simulink model "uz_dac_spi_interface"  (R2023a)
settings: Solver=FixedStepDiscrete  StartTime=0.0  StopTime=1000/100e6  RelTol=1e-3
libraries: hdlsllib x152, simulink x2
settings Model: DataTypeOverride=Off  Creator=ts  LastModifiedBy=ts
settings SolverCC: AlgebraicLoopSolver=TrustRegion
settings DataIOCC: LimitDataPoints=on  SaveOutput=off  SaveTime=off
settings OptimizationCC: BlockReduction=off  ConditionallyExecuteInputs=off  DefaultParameterBehavior=Inlined  LifeSpan=inf
settings DebuggingCC: AlgebraicLoopMsg=error  SingleTaskRateTransMsg=error  UnconnectedInputMsg=warning  UnconnectedOutputMsg=warning  UnconnectedLineMsg=warning  AllowSymbolicDim=off  StrictBusMsg=ErrorOnBusTreatedAsVector  SFUnexpectedBacktrackingDiag=warning  SFNoUnconditionalDefaultTransitionDiag=warning  SFExecutionAtInitializationDiag=none  ArithmeticOperatorsInVariantConditions=warning
settings HardwareCC: ProdBitPerPointer=32  ProdBitPerSizeT=32  ProdBitPerPtrDiffT=32  ProdLargestAtomicFloat=None  ProdIntDivRoundTo=Undefined  ProdEndianess=Unspecified  ProdWordSize=32  ProdHWDeviceType=ASIC/FPGA->ASIC/FPGA  ProdEqTarget=off
settings ModelReferenceCC: EnableRefExpFcnMdlSchedulingChecks=on
settings SFSimCC: SimUseLocalCustomCode=off  CustomCodeUndefinedFunction=UseInterfaceOnly
settings RTWCC: RTWUseLocalCustomCode=off
settings CodeAppCC: StateflowObjectComments=on
settings GRTTargetCC: TargetLangStandard=C89/C90 (ANSI)
settings ConfigComp: CovScope=ReferencedModels  CovMetricSettings=dw  CovSaveCumulativeToWorkspaceVar=on  CovSaveSingleToWorkspaceVar=on  CovExternalEMLEnable=off  CovSFcnEnable=off

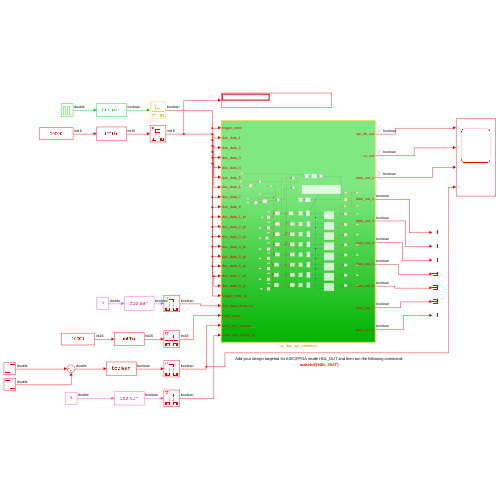
[thumbnail: Simulink's stored preview of the top-level diagram]
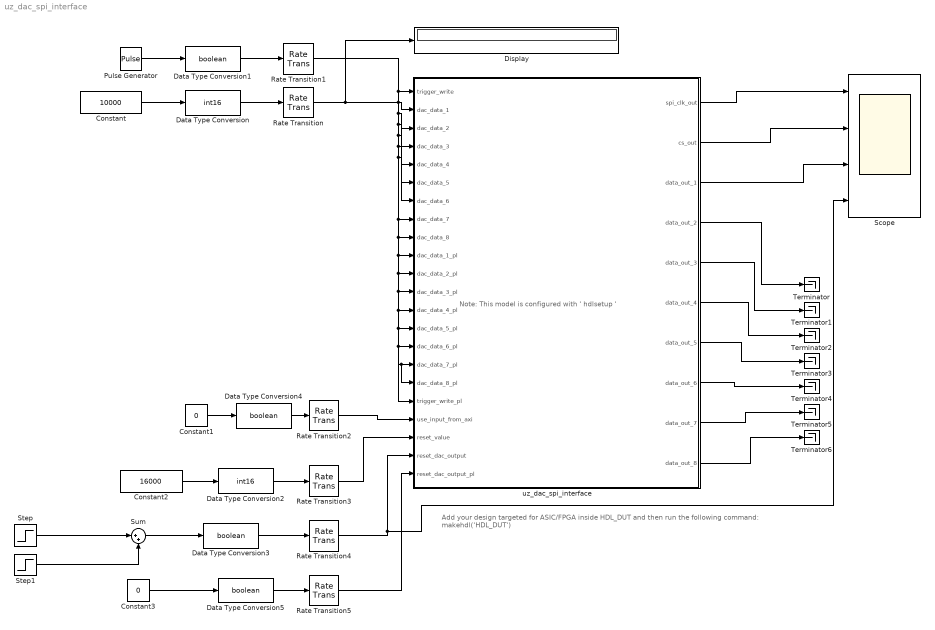
== system uz_dac_spi_interface ==
  note: Note: This model is configured with ' hdlsetup '
  note: Add your design targeted for ASIC/FPGA inside HDL_DUT and then run the following command:
      | makehdl('HDL_DUT')
  Constant : Constant  Value=10000  OutDataTypeStr=int16  SampleTime=1/100e6
  Constant1 : Constant  Value=0
  Constant2 : Constant  Value=16000  OutDataTypeStr=int16  SampleTime=1/100e6
  Constant3 : Constant  Value=0
  Data Type Conversion : DataTypeConversion  OutDataTypeStr=int16  SaturateOnIntegerOverflow=off  RndMeth=Floor
  Data Type Conversion{1,3..5} (4 alike) : DataTypeConversion  OutDataTypeStr=boolean  SaturateOnIntegerOverflow=off  RndMeth=Floor
  Data Type Conversion2 : DataTypeConversion  OutDataTypeStr=int16  SaturateOnIntegerOverflow=off  RndMeth=Floor
  Display : Display
      settings: Format=binary (Stored Integer)
  Pulse Generator : DiscretePulseGenerator  PulseType=Time based  Period=200/100e6  PulseWidth=10
  Rate Transition{,1..5} (6 alike) : RateTransition  OutPortSampleTime=1/100e6
  Scope : Scope  NumInputPorts=4
  Step : Step  Time=240/100e6
  Step1 : Step  Time=500/100e6  After=-1
  Sum : Sum  Inputs=|++
  Terminator{,1..6} (7 alike) : Terminator
  uz_dac_spi_interface : Subsystem  TreatAsAtomicUnit=on
  wires:
  Constant/1 -> Data Type Conversion/1
  uz_dac_spi_interface/3(data_out_1) -> Scope/3
  Data Type Conversion/1 -> Rate Transition/1
  Rate Transition/1 -> Display/1, uz_dac_spi_interface/17(dac_data_8_pl), uz_dac_spi_interface/16(dac_data_7_pl), uz_dac_spi_interface/15(dac_data_6_pl), uz_dac_spi_interface/14(dac_data_5_pl), uz_dac_spi_interface/13(dac_data_4_pl), uz_dac_spi_interface/12(dac_data_3_pl), uz_dac_spi_interface/11(dac_data_2_pl), uz_dac_spi_interface/10(dac_data_1_pl), uz_dac_spi_interface/9(dac_data_8), uz_dac_spi_interface/8(dac_data_7), uz_dac_spi_interface/7(dac_data_6), uz_dac_spi_interface/6(dac_data_5), uz_dac_spi_interface/5(dac_data_4), uz_dac_spi_interface/4(dac_data_3), uz_dac_spi_interface/3(dac_data_2), uz_dac_spi_interface/2(dac_data_1)
  uz_dac_spi_interface/2(cs_out) -> Scope/2
  uz_dac_spi_interface/1(spi_clk_out) -> Scope/1
  Rate Transition1/1 -> uz_dac_spi_interface/1(trigger_write), uz_dac_spi_interface/18(trigger_write_pl)
  Data Type Conversion1/1 -> Rate Transition1/1
  Pulse Generator/1 -> Data Type Conversion1/1
  Rate Transition2/1 -> uz_dac_spi_interface/19(use_input_from_axi)
  Constant1/1 -> Data Type Conversion4/1
  uz_dac_spi_interface/4(data_out_2) -> Terminator/1
  uz_dac_spi_interface/5(data_out_3) -> Terminator1/1
  uz_dac_spi_interface/6(data_out_4) -> Terminator2/1
  uz_dac_spi_interface/7(data_out_5) -> Terminator3/1
  uz_dac_spi_interface/8(data_out_6) -> Terminator4/1
  uz_dac_spi_interface/9(data_out_7) -> Terminator5/1
  uz_dac_spi_interface/10(data_out_8) -> Terminator6/1
  Constant2/1 -> Data Type Conversion2/1
  Data Type Conversion2/1 -> Rate Transition3/1
  Rate Transition3/1 -> uz_dac_spi_interface/20(reset_value)
  Data Type Conversion3/1 -> Rate Transition4/1
  Constant3/1 -> Data Type Conversion5/1
  Rate Transition5/1 -> uz_dac_spi_interface/22(reset_dac_output_pl)
  Data Type Conversion4/1 -> Rate Transition2/1
  Data Type Conversion5/1 -> Rate Transition5/1
  Rate Transition4/1 -> Scope/4, uz_dac_spi_interface/21(reset_dac_output)
  Sum/1 -> Data Type Conversion3/1
  Step/1 -> Sum/1
  Step1/1 -> Sum/2

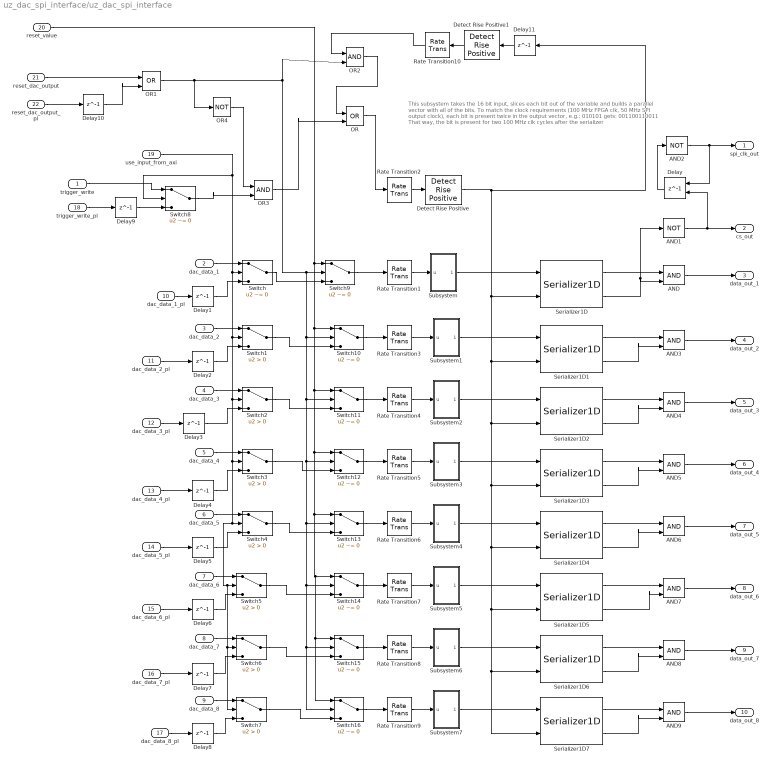
== system uz_dac_spi_interface/uz_dac_spi_interface ==
  note: This subsystem takes the 16 bit input, slices each bit out of the variable and builds a parallel vector with all of the bits.
      | To match the clock requirements (100 MHz FPGA clk, 50 MHz SPI output clock), each bit is present twice in the output vector, e.g.:
      | 010101 gets:
      | 001100110011
      | That way, the bit is present for two 100 MHz clk cycles after the serializer
  trigger_write : Inport
  dac_data_1 : Inport  Port=2
  dac_data_2 : Inport  Port=3
  dac_data_3 : Inport  Port=4
  dac_data_4 : Inport  Port=5
  dac_data_5 : Inport  Port=6
  dac_data_6 : Inport  Port=7
  dac_data_7 : Inport  Port=8
  dac_data_8 : Inport  Port=9
  dac_data_1_pl : Inport  Port=10
  dac_data_2_pl : Inport  Port=11
  dac_data_3_pl : Inport  Port=12
  dac_data_4_pl : Inport  Port=13
  dac_data_5_pl : Inport  Port=14
  dac_data_6_pl : Inport  Port=15
  dac_data_7_pl : Inport  Port=16
  dac_data_8_pl : Inport  Port=17
  trigger_write_pl : Inport  Port=18
  use_input_from_axi : Inport  Port=19
  reset_value : Inport  Port=20
  reset_dac_output : Inport  Port=21
  reset_dac_output_pl : Inport  Port=22
  AND{,3..9} (8 alike) : Logic  IconShape=distinctive  AllPortsSameDT=off  OutDataTypeStr=boolean
  AND1 : Logic  Operator=NOT  IconShape=distinctive  AllPortsSameDT=off  OutDataTypeStr=boolean
  AND2 : Logic  Operator=NOT  IconShape=distinctive  AllPortsSameDT=off  OutDataTypeStr=boolean
  Delay : Delay  DelayLength=1  InitialCondition=1  ExternalReset=Level
      settings: InputPortMap=u0,r5
  Delay{1..11} (11 alike) : Delay  DelayLength=1
  Detect Rise Positive : simulink/Logic and Bit Operations/Detect Rise Positive  vinit=0  OutDataTypeStr=boolean
  Detect Rise Positive1 : simulink/Logic and Bit Operations/Detect Rise Positive  vinit=0  OutDataTypeStr=boolean
  OR : Logic  Operator=OR  IconShape=distinctive  AllPortsSameDT=off  OutDataTypeStr=boolean
  OR1 : Logic  Operator=OR  IconShape=distinctive  AllPortsSameDT=off  OutDataTypeStr=boolean
  OR2 : Logic  IconShape=distinctive  AllPortsSameDT=off  OutDataTypeStr=boolean
  OR3 : Logic  IconShape=distinctive  AllPortsSameDT=off  OutDataTypeStr=boolean
  OR4 : Logic  Operator=NOT  IconShape=distinctive  AllPortsSameDT=off  OutDataTypeStr=boolean
  Rate Transition{1..9} (9 alike) : RateTransition  OutPortSampleTime=32/100e6
  Rate Transition10 : RateTransition
  Serializer1D{,1..7} (8 alike) : hdlsllib/HDL Operations/Serializer1D  Ratio=32  IdleCycles=0  validIn=on  startOut=off  validOut=on  inputDataDimensions=-1  inputSampleTime=-1  inputSignalType=auto
  Subsystem : Subsystem
  Subsystem1 : Subsystem
  Subsystem2 : Subsystem
  Subsystem3 : Subsystem
  Subsystem4 : Subsystem
  Subsystem5 : Subsystem
  Subsystem6 : Subsystem
  Subsystem7 : Subsystem
  Switch{,8..16} (10 alike) : Switch  Criteria=u2 ~= 0  SaturateOnIntegerOverflow=off  InputSameDT=off
  Switch{1..7} (7 alike) : Switch  Criteria=u2 > Threshold  SaturateOnIntegerOverflow=off  InputSameDT=off
  spi_clk_out : Outport
  cs_out : Outport  Port=2
  data_out_1 : Outport  Port=3  VectorParamsAs1DForOutWhenUnconnected=off
  data_out_2 : Outport  Port=4  VectorParamsAs1DForOutWhenUnconnected=off
  data_out_3 : Outport  Port=5  VectorParamsAs1DForOutWhenUnconnected=off
  data_out_4 : Outport  Port=6  VectorParamsAs1DForOutWhenUnconnected=off
  data_out_5 : Outport  Port=7  VectorParamsAs1DForOutWhenUnconnected=off
  data_out_6 : Outport  Port=8  VectorParamsAs1DForOutWhenUnconnected=off
  data_out_7 : Outport  Port=9  VectorParamsAs1DForOutWhenUnconnected=off
  data_out_8 : Outport  Port=10  VectorParamsAs1DForOutWhenUnconnected=off
  wires:
  AND/1 -> data_out_1/1
  Serializer1D/2 -> AND1/1, AND/2
  trigger_write/1 -> Switch8/1
  Detect Rise Positive/1 -> Serializer1D6/2, Serializer1D7/2, Serializer1D5/2, Serializer1D4/2, Serializer1D3/2, Serializer1D2/2, Serializer1D1/2, Serializer1D/2, Delay11/1
  Serializer1D/1 -> AND/1
  AND1/1 -> cs_out/1, Delay/2
  AND2/1 -> Delay/1, spi_clk_out/1
  Delay/1 -> AND2/1
  Rate Transition2/1 -> Detect Rise Positive/1
  Rate Transition1/1 -> Subsystem/1(u)
  Subsystem/1(Out1) -> Serializer1D/1
  Subsystem2/1(Out1) -> Serializer1D2/1
  Subsystem3/1(Out1) -> Serializer1D3/1
  Subsystem1/1(Out1) -> Serializer1D1/1
  Subsystem4/1(Out1) -> Serializer1D4/1
  Rate Transition3/1 -> Subsystem1/1(u)
  Rate Transition4/1 -> Subsystem2/1(u)
  Rate Transition5/1 -> Subsystem3/1(u)
  Rate Transition6/1 -> Subsystem4/1(u)
  Subsystem7/1(Out1) -> Serializer1D7/1
  Subsystem5/1(Out1) -> Serializer1D5/1
  Subsystem6/1(Out1) -> Serializer1D6/1
  Rate Transition7/1 -> Subsystem5/1(u)
  Rate Transition8/1 -> Subsystem6/1(u)
  Rate Transition9/1 -> Subsystem7/1(u)
  AND3/1 -> data_out_2/1
  Serializer1D1/1 -> AND3/1
  Serializer1D1/2 -> AND3/2
  AND4/1 -> data_out_3/1
  AND5/1 -> data_out_4/1
  AND6/1 -> data_out_5/1
  AND7/1 -> data_out_6/1
  AND8/1 -> data_out_7/1
  AND9/1 -> data_out_8/1
  Serializer1D2/1 -> AND4/1
  Serializer1D2/2 -> AND4/2
  Serializer1D3/1 -> AND5/1
  Serializer1D3/2 -> AND5/2
  Serializer1D4/1 -> AND6/1
  Serializer1D4/2 -> AND6/2
  Serializer1D5/1 -> AND7/1
  Serializer1D5/2 -> AND7/2
  Serializer1D6/1 -> AND8/1
  Serializer1D6/2 -> AND8/2
  Serializer1D7/1 -> AND9/1
  Serializer1D7/2 -> AND9/2
  dac_data_1/1 -> Switch/1
  dac_data_3/1 -> Switch2/1
  dac_data_2/1 -> Switch1/1
  dac_data_4/1 -> Switch3/1
  dac_data_5/1 -> Switch4/1
  dac_data_6/1 -> Switch5/1
  dac_data_7/1 -> Switch6/1
  dac_data_8/1 -> Switch7/1
  dac_data_1_pl/1 -> Delay1/1
  dac_data_2_pl/1 -> Delay2/1
  dac_data_3_pl/1 -> Delay3/1
  dac_data_4_pl/1 -> Delay4/1
  dac_data_5_pl/1 -> Delay5/1
  dac_data_6_pl/1 -> Delay6/1
  dac_data_7_pl/1 -> Delay7/1
  dac_data_8_pl/1 -> Delay8/1
  Delay1/1 -> Switch/3
  Delay2/1 -> Switch1/3
  Delay3/1 -> Switch2/3
  Delay4/1 -> Switch3/3
  Delay5/1 -> Switch4/3
  Delay6/1 -> Switch5/3
  Delay7/1 -> Switch6/3
  Delay8/1 -> Switch7/3
  trigger_write_pl/1 -> Delay9/1
  Delay9/1 -> Switch8/3
  use_input_from_axi/1 -> Switch7/2, Switch6/2, Switch5/2, Switch4/2, Switch3/2, Switch2/2, Switch1/2, Switch/2, Switch8/2
  Switch9/1 -> Rate Transition1/1
  Switch10/1 -> Rate Transition3/1
  Switch11/1 -> Rate Transition4/1
  Switch12/1 -> Rate Transition5/1
  Switch13/1 -> Rate Transition6/1
  Switch14/1 -> Rate Transition7/1
  Switch15/1 -> Rate Transition8/1
  Switch16/1 -> Rate Transition9/1
  OR/1 -> Rate Transition2/1
  reset_dac_output_pl/1 -> Delay10/1
  OR1/1 -> OR4/1, OR2/2, Switch16/2, Switch15/2, Switch14/2, Switch13/2, Switch12/2, Switch11/2, Switch10/2, Switch9/2
  reset_dac_output/1 -> OR1/1
  Delay10/1 -> OR1/2
  reset_value/1 -> Switch16/1, Switch15/1, Switch14/1, Switch13/1, Switch12/1, Switch11/1, Switch10/1, Switch9/1
  Switch/1 -> Switch9/3
  Switch1/1 -> Switch10/3
  Switch2/1 -> Switch11/3
  Switch3/1 -> Switch12/3
  Switch4/1 -> Switch13/3
  Switch5/1 -> Switch14/3
  Switch6/1 -> Switch15/3
  Switch7/1 -> Switch16/3
  OR2/1 -> OR/1
  Detect Rise Positive1/1 -> Rate Transition10/1
  Rate Transition10/1 -> OR2/1
  Delay11/1 -> Detect Rise Positive1/1
  Switch8/1 -> OR3/2
  OR3/1 -> OR/2
  OR4/1 -> OR3/1

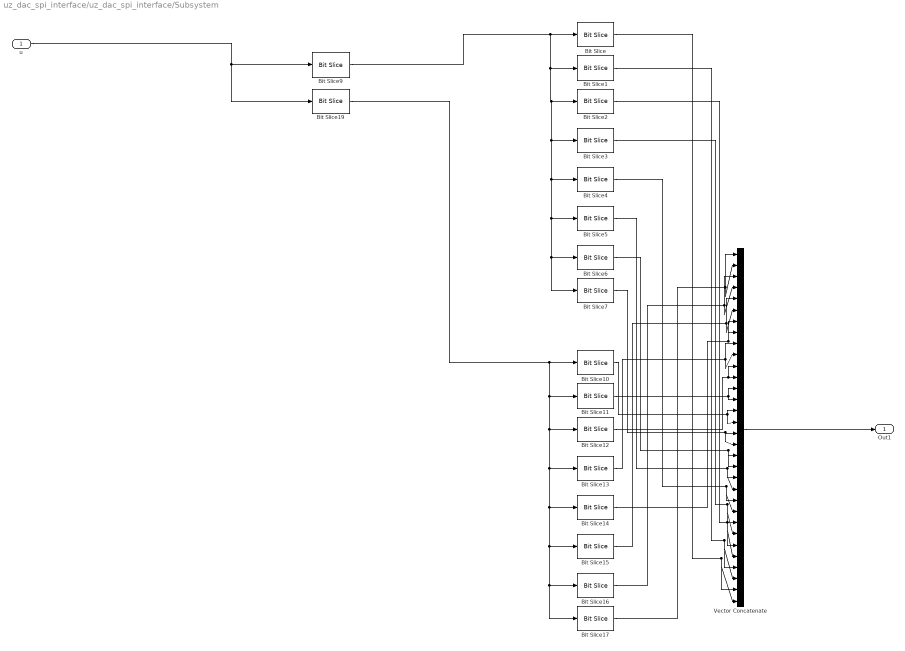
== system uz_dac_spi_interface/uz_dac_spi_interface/Subsystem ==
  u : Inport
  Bit Slice : hdlsllib/Logic and Bit Operations/Bit Slice  lidx=0  ridx=0
  Bit Slice1 : hdlsllib/Logic and Bit Operations/Bit Slice  lidx=1  ridx=1
  Bit Slice10 : hdlsllib/Logic and Bit Operations/Bit Slice  lidx=0  ridx=0
  Bit Slice11 : hdlsllib/Logic and Bit Operations/Bit Slice  lidx=1  ridx=1
  Bit Slice12 : hdlsllib/Logic and Bit Operations/Bit Slice  lidx=2  ridx=2
  Bit Slice13 : hdlsllib/Logic and Bit Operations/Bit Slice  lidx=3  ridx=3
  Bit Slice14 : hdlsllib/Logic and Bit Operations/Bit Slice  lidx=4  ridx=4
  Bit Slice15 : hdlsllib/Logic and Bit Operations/Bit Slice  lidx=5  ridx=5
  Bit Slice16 : hdlsllib/Logic and Bit Operations/Bit Slice  lidx=6  ridx=6
  Bit Slice17 : hdlsllib/Logic and Bit Operations/Bit Slice  lidx=7  ridx=7
  Bit Slice19 : hdlsllib/Logic and Bit Operations/Bit Slice  lidx=15  ridx=8
  Bit Slice2 : hdlsllib/Logic and Bit Operations/Bit Slice  lidx=2  ridx=2
  Bit Slice3 : hdlsllib/Logic and Bit Operations/Bit Slice  lidx=3  ridx=3
  Bit Slice4 : hdlsllib/Logic and Bit Operations/Bit Slice  lidx=4  ridx=4
  Bit Slice5 : hdlsllib/Logic and Bit Operations/Bit Slice  lidx=5  ridx=5
  Bit Slice6 : hdlsllib/Logic and Bit Operations/Bit Slice  lidx=6  ridx=6
  Bit Slice7 : hdlsllib/Logic and Bit Operations/Bit Slice  lidx=7  ridx=7
  Bit Slice9 : hdlsllib/Logic and Bit Operations/Bit Slice  lidx=7  ridx=0
  Vector Concatenate : Concatenate  NumInputs=32
  Out1 : Outport
  wires:
  Bit Slice10/1 -> Vector Concatenate/16, Vector Concatenate/15
  Bit Slice4/1 -> Vector Concatenate/24, Vector Concatenate/23
  Bit Slice6/1 -> Vector Concatenate/20, Vector Concatenate/19
  Bit Slice5/1 -> Vector Concatenate/22, Vector Concatenate/21
  u/1 -> Bit Slice19/1, Bit Slice9/1
  Bit Slice19/1 -> Bit Slice17/1, Bit Slice16/1, Bit Slice15/1, Bit Slice14/1, Bit Slice13/1, Bit Slice12/1, Bit Slice11/1, Bit Slice10/1
  Bit Slice11/1 -> Vector Concatenate/14, Vector Concatenate/13
  Bit Slice9/1 -> Bit Slice7/1, Bit Slice6/1, Bit Slice5/1, Bit Slice4/1, Bit Slice3/1, Bit Slice2/1, Bit Slice1/1, Bit Slice/1
  Bit Slice13/1 -> Vector Concatenate/10, Vector Concatenate/9
  Vector Concatenate/1 -> Out1/1
  Bit Slice7/1 -> Vector Concatenate/18, Vector Concatenate/17
  Bit Slice1/1 -> Vector Concatenate/30, Vector Concatenate/29
  Bit Slice/1 -> Vector Concatenate/32, Vector Concatenate/31
  Bit Slice17/1 -> Vector Concatenate/2, Vector Concatenate/1
  Bit Slice2/1 -> Vector Concatenate/28, Vector Concatenate/27
  Bit Slice12/1 -> Vector Concatenate/12, Vector Concatenate/11
  Bit Slice16/1 -> Vector Concatenate/4, Vector Concatenate/3
  Bit Slice14/1 -> Vector Concatenate/8, Vector Concatenate/7
  Bit Slice3/1 -> Vector Concatenate/26, Vector Concatenate/25
  Bit Slice15/1 -> Vector Concatenate/6, Vector Concatenate/5

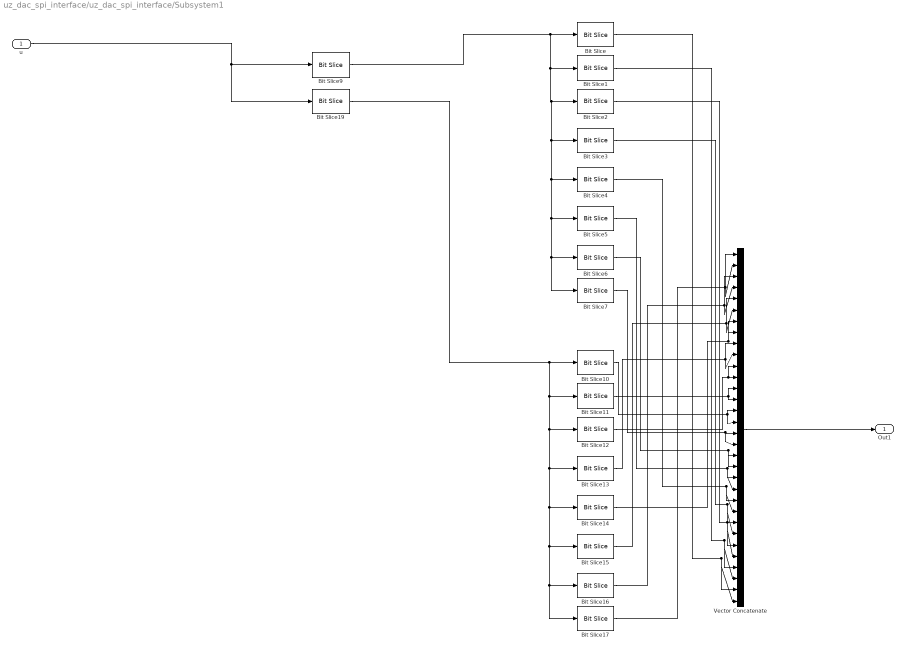
== system uz_dac_spi_interface/uz_dac_spi_interface/Subsystem1 ==
  u : Inport
  Bit Slice : hdlsllib/Logic and Bit Operations/Bit Slice  lidx=0  ridx=0
  Bit Slice1 : hdlsllib/Logic and Bit Operations/Bit Slice  lidx=1  ridx=1
  Bit Slice10 : hdlsllib/Logic and Bit Operations/Bit Slice  lidx=0  ridx=0
  Bit Slice11 : hdlsllib/Logic and Bit Operations/Bit Slice  lidx=1  ridx=1
  Bit Slice12 : hdlsllib/Logic and Bit Operations/Bit Slice  lidx=2  ridx=2
  Bit Slice13 : hdlsllib/Logic and Bit Operations/Bit Slice  lidx=3  ridx=3
  Bit Slice14 : hdlsllib/Logic and Bit Operations/Bit Slice  lidx=4  ridx=4
  Bit Slice15 : hdlsllib/Logic and Bit Operations/Bit Slice  lidx=5  ridx=5
  Bit Slice16 : hdlsllib/Logic and Bit Operations/Bit Slice  lidx=6  ridx=6
  Bit Slice17 : hdlsllib/Logic and Bit Operations/Bit Slice  lidx=7  ridx=7
  Bit Slice19 : hdlsllib/Logic and Bit Operations/Bit Slice  lidx=15  ridx=8
  Bit Slice2 : hdlsllib/Logic and Bit Operations/Bit Slice  lidx=2  ridx=2
  Bit Slice3 : hdlsllib/Logic and Bit Operations/Bit Slice  lidx=3  ridx=3
  Bit Slice4 : hdlsllib/Logic and Bit Operations/Bit Slice  lidx=4  ridx=4
  Bit Slice5 : hdlsllib/Logic and Bit Operations/Bit Slice  lidx=5  ridx=5
  Bit Slice6 : hdlsllib/Logic and Bit Operations/Bit Slice  lidx=6  ridx=6
  Bit Slice7 : hdlsllib/Logic and Bit Operations/Bit Slice  lidx=7  ridx=7
  Bit Slice9 : hdlsllib/Logic and Bit Operations/Bit Slice  lidx=7  ridx=0
  Vector Concatenate : Concatenate  NumInputs=32
  Out1 : Outport
  wires:
  Bit Slice15/1 -> Vector Concatenate/5, Vector Concatenate/6
  Bit Slice3/1 -> Vector Concatenate/25, Vector Concatenate/26
  Bit Slice14/1 -> Vector Concatenate/7, Vector Concatenate/8
  Bit Slice16/1 -> Vector Concatenate/3, Vector Concatenate/4
  Bit Slice12/1 -> Vector Concatenate/11, Vector Concatenate/12
  Bit Slice2/1 -> Vector Concatenate/27, Vector Concatenate/28
  Bit Slice17/1 -> Vector Concatenate/1, Vector Concatenate/2
  Bit Slice/1 -> Vector Concatenate/31, Vector Concatenate/32
  Bit Slice1/1 -> Vector Concatenate/29, Vector Concatenate/30
  Bit Slice7/1 -> Vector Concatenate/17, Vector Concatenate/18
  Vector Concatenate/1 -> Out1/1
  Bit Slice13/1 -> Vector Concatenate/9, Vector Concatenate/10
  Bit Slice9/1 -> Bit Slice/1, Bit Slice1/1, Bit Slice2/1, Bit Slice3/1, Bit Slice4/1, Bit Slice5/1, Bit Slice6/1, Bit Slice7/1
  Bit Slice11/1 -> Vector Concatenate/13, Vector Concatenate/14
  Bit Slice19/1 -> Bit Slice10/1, Bit Slice11/1, Bit Slice12/1, Bit Slice13/1, Bit Slice14/1, Bit Slice15/1, Bit Slice16/1, Bit Slice17/1
  u/1 -> Bit Slice9/1, Bit Slice19/1
  Bit Slice5/1 -> Vector Concatenate/21, Vector Concatenate/22
  Bit Slice6/1 -> Vector Concatenate/19, Vector Concatenate/20
  Bit Slice4/1 -> Vector Concatenate/23, Vector Concatenate/24
  Bit Slice10/1 -> Vector Concatenate/15, Vector Concatenate/16

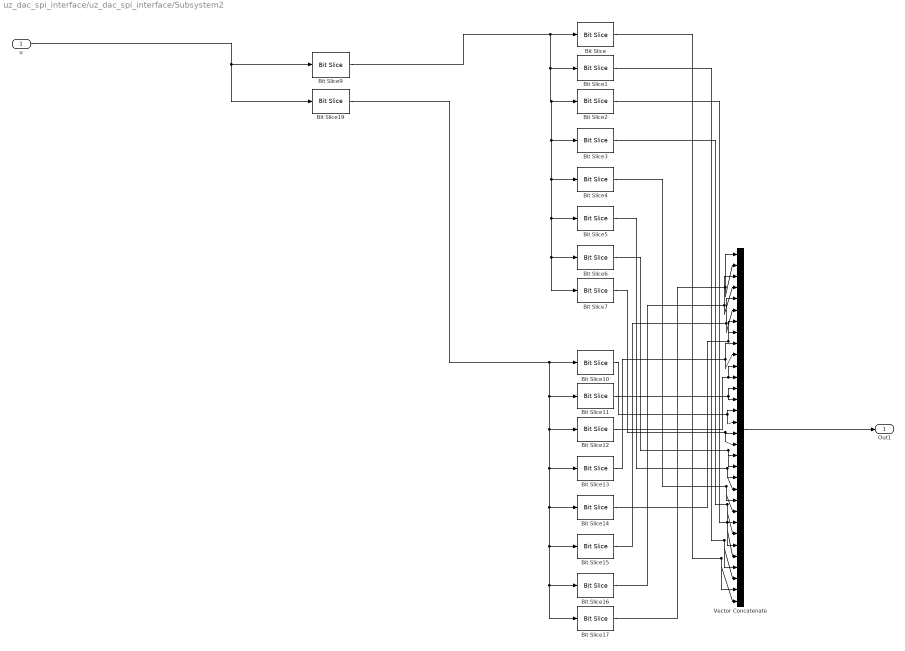
== system uz_dac_spi_interface/uz_dac_spi_interface/Subsystem2 ==
  u : Inport
  Bit Slice : hdlsllib/Logic and Bit Operations/Bit Slice  lidx=0  ridx=0
  Bit Slice1 : hdlsllib/Logic and Bit Operations/Bit Slice  lidx=1  ridx=1
  Bit Slice10 : hdlsllib/Logic and Bit Operations/Bit Slice  lidx=0  ridx=0
  Bit Slice11 : hdlsllib/Logic and Bit Operations/Bit Slice  lidx=1  ridx=1
  Bit Slice12 : hdlsllib/Logic and Bit Operations/Bit Slice  lidx=2  ridx=2
  Bit Slice13 : hdlsllib/Logic and Bit Operations/Bit Slice  lidx=3  ridx=3
  Bit Slice14 : hdlsllib/Logic and Bit Operations/Bit Slice  lidx=4  ridx=4
  Bit Slice15 : hdlsllib/Logic and Bit Operations/Bit Slice  lidx=5  ridx=5
  Bit Slice16 : hdlsllib/Logic and Bit Operations/Bit Slice  lidx=6  ridx=6
  Bit Slice17 : hdlsllib/Logic and Bit Operations/Bit Slice  lidx=7  ridx=7
  Bit Slice19 : hdlsllib/Logic and Bit Operations/Bit Slice  lidx=15  ridx=8
  Bit Slice2 : hdlsllib/Logic and Bit Operations/Bit Slice  lidx=2  ridx=2
  Bit Slice3 : hdlsllib/Logic and Bit Operations/Bit Slice  lidx=3  ridx=3
  Bit Slice4 : hdlsllib/Logic and Bit Operations/Bit Slice  lidx=4  ridx=4
  Bit Slice5 : hdlsllib/Logic and Bit Operations/Bit Slice  lidx=5  ridx=5
  Bit Slice6 : hdlsllib/Logic and Bit Operations/Bit Slice  lidx=6  ridx=6
  Bit Slice7 : hdlsllib/Logic and Bit Operations/Bit Slice  lidx=7  ridx=7
  Bit Slice9 : hdlsllib/Logic and Bit Operations/Bit Slice  lidx=7  ridx=0
  Vector Concatenate : Concatenate  NumInputs=32
  Out1 : Outport
  wires:
  Bit Slice10/1 -> Vector Concatenate/16, Vector Concatenate/15
  Bit Slice4/1 -> Vector Concatenate/24, Vector Concatenate/23
  Bit Slice6/1 -> Vector Concatenate/20, Vector Concatenate/19
  Bit Slice5/1 -> Vector Concatenate/22, Vector Concatenate/21
  u/1 -> Bit Slice19/1, Bit Slice9/1
  Bit Slice19/1 -> Bit Slice17/1, Bit Slice16/1, Bit Slice15/1, Bit Slice14/1, Bit Slice13/1, Bit Slice12/1, Bit Slice11/1, Bit Slice10/1
  Bit Slice11/1 -> Vector Concatenate/14, Vector Concatenate/13
  Bit Slice9/1 -> Bit Slice7/1, Bit Slice6/1, Bit Slice5/1, Bit Slice4/1, Bit Slice3/1, Bit Slice2/1, Bit Slice1/1, Bit Slice/1
  Bit Slice13/1 -> Vector Concatenate/10, Vector Concatenate/9
  Vector Concatenate/1 -> Out1/1
  Bit Slice7/1 -> Vector Concatenate/18, Vector Concatenate/17
  Bit Slice1/1 -> Vector Concatenate/30, Vector Concatenate/29
  Bit Slice/1 -> Vector Concatenate/32, Vector Concatenate/31
  Bit Slice17/1 -> Vector Concatenate/2, Vector Concatenate/1
  Bit Slice2/1 -> Vector Concatenate/28, Vector Concatenate/27
  Bit Slice12/1 -> Vector Concatenate/12, Vector Concatenate/11
  Bit Slice16/1 -> Vector Concatenate/4, Vector Concatenate/3
  Bit Slice14/1 -> Vector Concatenate/8, Vector Concatenate/7
  Bit Slice3/1 -> Vector Concatenate/26, Vector Concatenate/25
  Bit Slice15/1 -> Vector Concatenate/6, Vector Concatenate/5

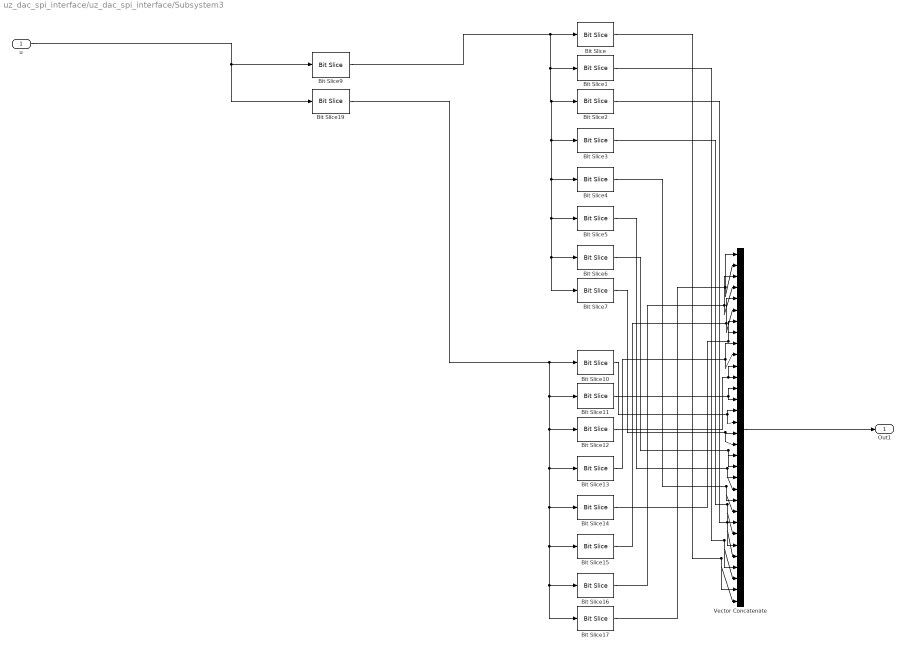
== system uz_dac_spi_interface/uz_dac_spi_interface/Subsystem3 ==
  u : Inport
  Bit Slice : hdlsllib/Logic and Bit Operations/Bit Slice  lidx=0  ridx=0
  Bit Slice1 : hdlsllib/Logic and Bit Operations/Bit Slice  lidx=1  ridx=1
  Bit Slice10 : hdlsllib/Logic and Bit Operations/Bit Slice  lidx=0  ridx=0
  Bit Slice11 : hdlsllib/Logic and Bit Operations/Bit Slice  lidx=1  ridx=1
  Bit Slice12 : hdlsllib/Logic and Bit Operations/Bit Slice  lidx=2  ridx=2
  Bit Slice13 : hdlsllib/Logic and Bit Operations/Bit Slice  lidx=3  ridx=3
  Bit Slice14 : hdlsllib/Logic and Bit Operations/Bit Slice  lidx=4  ridx=4
  Bit Slice15 : hdlsllib/Logic and Bit Operations/Bit Slice  lidx=5  ridx=5
  Bit Slice16 : hdlsllib/Logic and Bit Operations/Bit Slice  lidx=6  ridx=6
  Bit Slice17 : hdlsllib/Logic and Bit Operations/Bit Slice  lidx=7  ridx=7
  Bit Slice19 : hdlsllib/Logic and Bit Operations/Bit Slice  lidx=15  ridx=8
  Bit Slice2 : hdlsllib/Logic and Bit Operations/Bit Slice  lidx=2  ridx=2
  Bit Slice3 : hdlsllib/Logic and Bit Operations/Bit Slice  lidx=3  ridx=3
  Bit Slice4 : hdlsllib/Logic and Bit Operations/Bit Slice  lidx=4  ridx=4
  Bit Slice5 : hdlsllib/Logic and Bit Operations/Bit Slice  lidx=5  ridx=5
  Bit Slice6 : hdlsllib/Logic and Bit Operations/Bit Slice  lidx=6  ridx=6
  Bit Slice7 : hdlsllib/Logic and Bit Operations/Bit Slice  lidx=7  ridx=7
  Bit Slice9 : hdlsllib/Logic and Bit Operations/Bit Slice  lidx=7  ridx=0
  Vector Concatenate : Concatenate  NumInputs=32
  Out1 : Outport
  wires:
  Bit Slice15/1 -> Vector Concatenate/5, Vector Concatenate/6
  Bit Slice3/1 -> Vector Concatenate/25, Vector Concatenate/26
  Bit Slice14/1 -> Vector Concatenate/7, Vector Concatenate/8
  Bit Slice16/1 -> Vector Concatenate/3, Vector Concatenate/4
  Bit Slice12/1 -> Vector Concatenate/11, Vector Concatenate/12
  Bit Slice2/1 -> Vector Concatenate/27, Vector Concatenate/28
  Bit Slice17/1 -> Vector Concatenate/1, Vector Concatenate/2
  Bit Slice/1 -> Vector Concatenate/31, Vector Concatenate/32
  Bit Slice1/1 -> Vector Concatenate/29, Vector Concatenate/30
  Bit Slice7/1 -> Vector Concatenate/17, Vector Concatenate/18
  Vector Concatenate/1 -> Out1/1
  Bit Slice13/1 -> Vector Concatenate/9, Vector Concatenate/10
  Bit Slice9/1 -> Bit Slice/1, Bit Slice1/1, Bit Slice2/1, Bit Slice3/1, Bit Slice4/1, Bit Slice5/1, Bit Slice6/1, Bit Slice7/1
  Bit Slice11/1 -> Vector Concatenate/13, Vector Concatenate/14
  Bit Slice19/1 -> Bit Slice10/1, Bit Slice11/1, Bit Slice12/1, Bit Slice13/1, Bit Slice14/1, Bit Slice15/1, Bit Slice16/1, Bit Slice17/1
  u/1 -> Bit Slice9/1, Bit Slice19/1
  Bit Slice5/1 -> Vector Concatenate/21, Vector Concatenate/22
  Bit Slice6/1 -> Vector Concatenate/19, Vector Concatenate/20
  Bit Slice4/1 -> Vector Concatenate/23, Vector Concatenate/24
  Bit Slice10/1 -> Vector Concatenate/15, Vector Concatenate/16

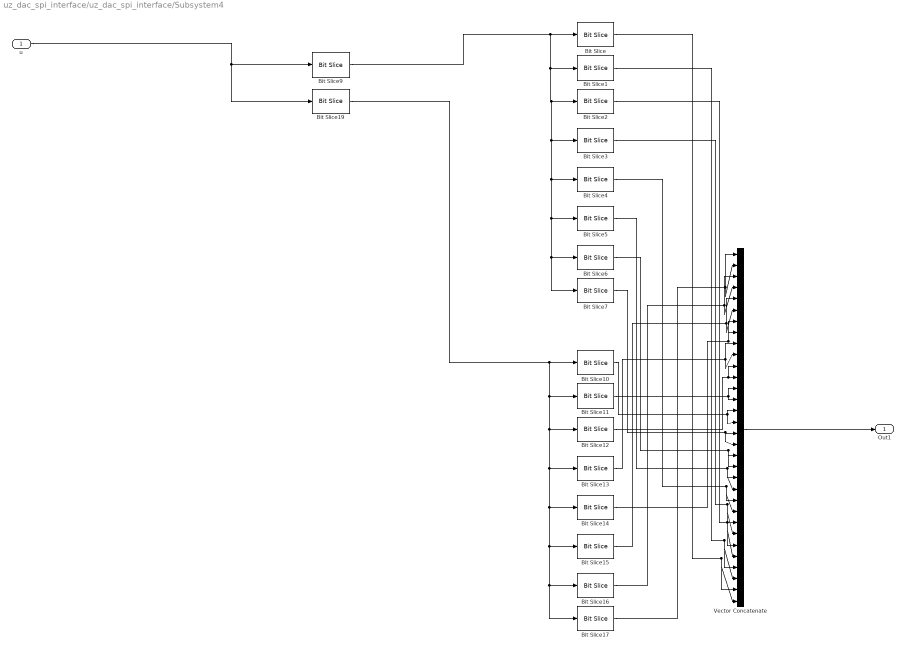
== system uz_dac_spi_interface/uz_dac_spi_interface/Subsystem4 ==
  u : Inport
  Bit Slice : hdlsllib/Logic and Bit Operations/Bit Slice  lidx=0  ridx=0
  Bit Slice1 : hdlsllib/Logic and Bit Operations/Bit Slice  lidx=1  ridx=1
  Bit Slice10 : hdlsllib/Logic and Bit Operations/Bit Slice  lidx=0  ridx=0
  Bit Slice11 : hdlsllib/Logic and Bit Operations/Bit Slice  lidx=1  ridx=1
  Bit Slice12 : hdlsllib/Logic and Bit Operations/Bit Slice  lidx=2  ridx=2
  Bit Slice13 : hdlsllib/Logic and Bit Operations/Bit Slice  lidx=3  ridx=3
  Bit Slice14 : hdlsllib/Logic and Bit Operations/Bit Slice  lidx=4  ridx=4
  Bit Slice15 : hdlsllib/Logic and Bit Operations/Bit Slice  lidx=5  ridx=5
  Bit Slice16 : hdlsllib/Logic and Bit Operations/Bit Slice  lidx=6  ridx=6
  Bit Slice17 : hdlsllib/Logic and Bit Operations/Bit Slice  lidx=7  ridx=7
  Bit Slice19 : hdlsllib/Logic and Bit Operations/Bit Slice  lidx=15  ridx=8
  Bit Slice2 : hdlsllib/Logic and Bit Operations/Bit Slice  lidx=2  ridx=2
  Bit Slice3 : hdlsllib/Logic and Bit Operations/Bit Slice  lidx=3  ridx=3
  Bit Slice4 : hdlsllib/Logic and Bit Operations/Bit Slice  lidx=4  ridx=4
  Bit Slice5 : hdlsllib/Logic and Bit Operations/Bit Slice  lidx=5  ridx=5
  Bit Slice6 : hdlsllib/Logic and Bit Operations/Bit Slice  lidx=6  ridx=6
  Bit Slice7 : hdlsllib/Logic and Bit Operations/Bit Slice  lidx=7  ridx=7
  Bit Slice9 : hdlsllib/Logic and Bit Operations/Bit Slice  lidx=7  ridx=0
  Vector Concatenate : Concatenate  NumInputs=32
  Out1 : Outport
  wires:
  Bit Slice15/1 -> Vector Concatenate/5, Vector Concatenate/6
  Bit Slice3/1 -> Vector Concatenate/25, Vector Concatenate/26
  Bit Slice14/1 -> Vector Concatenate/7, Vector Concatenate/8
  Bit Slice16/1 -> Vector Concatenate/3, Vector Concatenate/4
  Bit Slice12/1 -> Vector Concatenate/11, Vector Concatenate/12
  Bit Slice2/1 -> Vector Concatenate/27, Vector Concatenate/28
  Bit Slice17/1 -> Vector Concatenate/1, Vector Concatenate/2
  Bit Slice/1 -> Vector Concatenate/31, Vector Concatenate/32
  Bit Slice1/1 -> Vector Concatenate/29, Vector Concatenate/30
  Bit Slice7/1 -> Vector Concatenate/17, Vector Concatenate/18
  Vector Concatenate/1 -> Out1/1
  Bit Slice13/1 -> Vector Concatenate/9, Vector Concatenate/10
  Bit Slice9/1 -> Bit Slice/1, Bit Slice1/1, Bit Slice2/1, Bit Slice3/1, Bit Slice4/1, Bit Slice5/1, Bit Slice6/1, Bit Slice7/1
  Bit Slice11/1 -> Vector Concatenate/13, Vector Concatenate/14
  Bit Slice19/1 -> Bit Slice10/1, Bit Slice11/1, Bit Slice12/1, Bit Slice13/1, Bit Slice14/1, Bit Slice15/1, Bit Slice16/1, Bit Slice17/1
  u/1 -> Bit Slice9/1, Bit Slice19/1
  Bit Slice5/1 -> Vector Concatenate/21, Vector Concatenate/22
  Bit Slice6/1 -> Vector Concatenate/19, Vector Concatenate/20
  Bit Slice4/1 -> Vector Concatenate/23, Vector Concatenate/24
  Bit Slice10/1 -> Vector Concatenate/15, Vector Concatenate/16

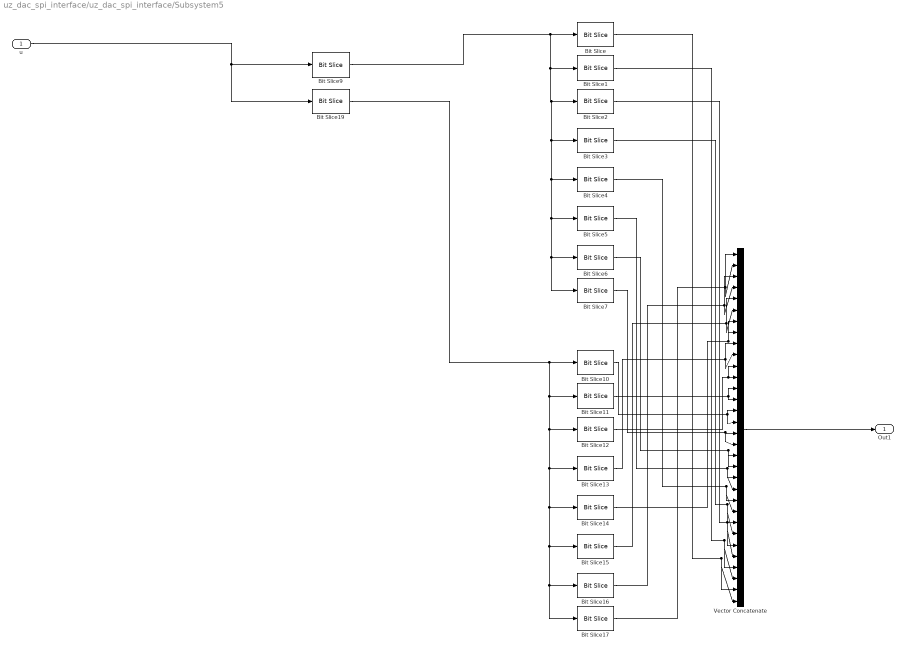
== system uz_dac_spi_interface/uz_dac_spi_interface/Subsystem5 ==
  u : Inport
  Bit Slice : hdlsllib/Logic and Bit Operations/Bit Slice  lidx=0  ridx=0
  Bit Slice1 : hdlsllib/Logic and Bit Operations/Bit Slice  lidx=1  ridx=1
  Bit Slice10 : hdlsllib/Logic and Bit Operations/Bit Slice  lidx=0  ridx=0
  Bit Slice11 : hdlsllib/Logic and Bit Operations/Bit Slice  lidx=1  ridx=1
  Bit Slice12 : hdlsllib/Logic and Bit Operations/Bit Slice  lidx=2  ridx=2
  Bit Slice13 : hdlsllib/Logic and Bit Operations/Bit Slice  lidx=3  ridx=3
  Bit Slice14 : hdlsllib/Logic and Bit Operations/Bit Slice  lidx=4  ridx=4
  Bit Slice15 : hdlsllib/Logic and Bit Operations/Bit Slice  lidx=5  ridx=5
  Bit Slice16 : hdlsllib/Logic and Bit Operations/Bit Slice  lidx=6  ridx=6
  Bit Slice17 : hdlsllib/Logic and Bit Operations/Bit Slice  lidx=7  ridx=7
  Bit Slice19 : hdlsllib/Logic and Bit Operations/Bit Slice  lidx=15  ridx=8
  Bit Slice2 : hdlsllib/Logic and Bit Operations/Bit Slice  lidx=2  ridx=2
  Bit Slice3 : hdlsllib/Logic and Bit Operations/Bit Slice  lidx=3  ridx=3
  Bit Slice4 : hdlsllib/Logic and Bit Operations/Bit Slice  lidx=4  ridx=4
  Bit Slice5 : hdlsllib/Logic and Bit Operations/Bit Slice  lidx=5  ridx=5
  Bit Slice6 : hdlsllib/Logic and Bit Operations/Bit Slice  lidx=6  ridx=6
  Bit Slice7 : hdlsllib/Logic and Bit Operations/Bit Slice  lidx=7  ridx=7
  Bit Slice9 : hdlsllib/Logic and Bit Operations/Bit Slice  lidx=7  ridx=0
  Vector Concatenate : Concatenate  NumInputs=32
  Out1 : Outport
  wires:
  Bit Slice10/1 -> Vector Concatenate/16, Vector Concatenate/15
  Bit Slice4/1 -> Vector Concatenate/24, Vector Concatenate/23
  Bit Slice6/1 -> Vector Concatenate/20, Vector Concatenate/19
  Bit Slice5/1 -> Vector Concatenate/22, Vector Concatenate/21
  u/1 -> Bit Slice19/1, Bit Slice9/1
  Bit Slice19/1 -> Bit Slice17/1, Bit Slice16/1, Bit Slice15/1, Bit Slice14/1, Bit Slice13/1, Bit Slice12/1, Bit Slice11/1, Bit Slice10/1
  Bit Slice11/1 -> Vector Concatenate/14, Vector Concatenate/13
  Bit Slice9/1 -> Bit Slice7/1, Bit Slice6/1, Bit Slice5/1, Bit Slice4/1, Bit Slice3/1, Bit Slice2/1, Bit Slice1/1, Bit Slice/1
  Bit Slice13/1 -> Vector Concatenate/10, Vector Concatenate/9
  Vector Concatenate/1 -> Out1/1
  Bit Slice7/1 -> Vector Concatenate/18, Vector Concatenate/17
  Bit Slice1/1 -> Vector Concatenate/30, Vector Concatenate/29
  Bit Slice/1 -> Vector Concatenate/32, Vector Concatenate/31
  Bit Slice17/1 -> Vector Concatenate/2, Vector Concatenate/1
  Bit Slice2/1 -> Vector Concatenate/28, Vector Concatenate/27
  Bit Slice12/1 -> Vector Concatenate/12, Vector Concatenate/11
  Bit Slice16/1 -> Vector Concatenate/4, Vector Concatenate/3
  Bit Slice14/1 -> Vector Concatenate/8, Vector Concatenate/7
  Bit Slice3/1 -> Vector Concatenate/26, Vector Concatenate/25
  Bit Slice15/1 -> Vector Concatenate/6, Vector Concatenate/5

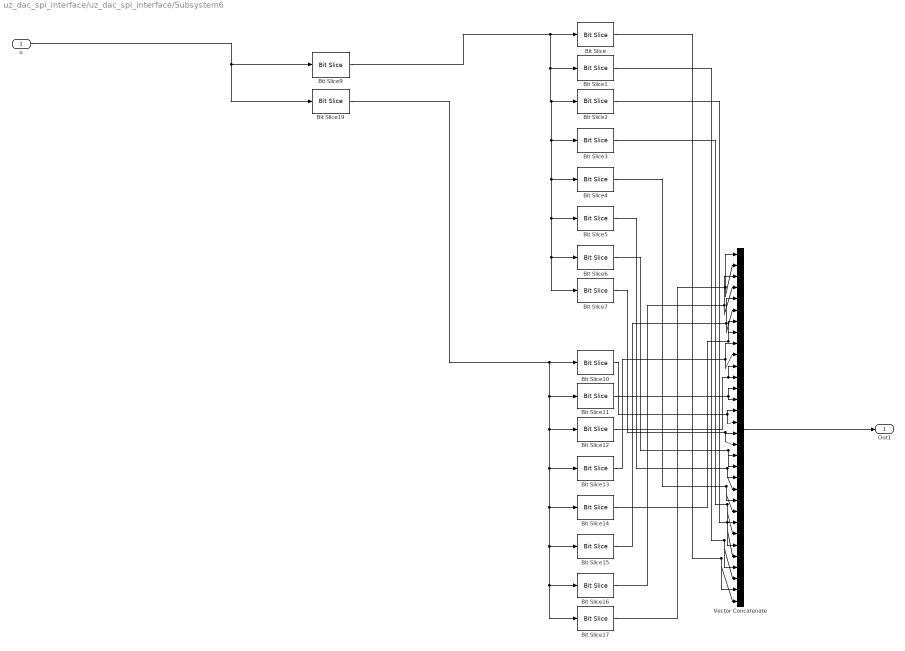
== system uz_dac_spi_interface/uz_dac_spi_interface/Subsystem6 ==
  u : Inport
  Bit Slice : hdlsllib/Logic and Bit Operations/Bit Slice  lidx=0  ridx=0
  Bit Slice1 : hdlsllib/Logic and Bit Operations/Bit Slice  lidx=1  ridx=1
  Bit Slice10 : hdlsllib/Logic and Bit Operations/Bit Slice  lidx=0  ridx=0
  Bit Slice11 : hdlsllib/Logic and Bit Operations/Bit Slice  lidx=1  ridx=1
  Bit Slice12 : hdlsllib/Logic and Bit Operations/Bit Slice  lidx=2  ridx=2
  Bit Slice13 : hdlsllib/Logic and Bit Operations/Bit Slice  lidx=3  ridx=3
  Bit Slice14 : hdlsllib/Logic and Bit Operations/Bit Slice  lidx=4  ridx=4
  Bit Slice15 : hdlsllib/Logic and Bit Operations/Bit Slice  lidx=5  ridx=5
  Bit Slice16 : hdlsllib/Logic and Bit Operations/Bit Slice  lidx=6  ridx=6
  Bit Slice17 : hdlsllib/Logic and Bit Operations/Bit Slice  lidx=7  ridx=7
  Bit Slice19 : hdlsllib/Logic and Bit Operations/Bit Slice  lidx=15  ridx=8
  Bit Slice2 : hdlsllib/Logic and Bit Operations/Bit Slice  lidx=2  ridx=2
  Bit Slice3 : hdlsllib/Logic and Bit Operations/Bit Slice  lidx=3  ridx=3
  Bit Slice4 : hdlsllib/Logic and Bit Operations/Bit Slice  lidx=4  ridx=4
  Bit Slice5 : hdlsllib/Logic and Bit Operations/Bit Slice  lidx=5  ridx=5
  Bit Slice6 : hdlsllib/Logic and Bit Operations/Bit Slice  lidx=6  ridx=6
  Bit Slice7 : hdlsllib/Logic and Bit Operations/Bit Slice  lidx=7  ridx=7
  Bit Slice9 : hdlsllib/Logic and Bit Operations/Bit Slice  lidx=7  ridx=0
  Vector Concatenate : Concatenate  NumInputs=32
  Out1 : Outport
  wires:
  Bit Slice15/1 -> Vector Concatenate/5, Vector Concatenate/6
  Bit Slice3/1 -> Vector Concatenate/25, Vector Concatenate/26
  Bit Slice14/1 -> Vector Concatenate/7, Vector Concatenate/8
  Bit Slice16/1 -> Vector Concatenate/3, Vector Concatenate/4
  Bit Slice12/1 -> Vector Concatenate/11, Vector Concatenate/12
  Bit Slice2/1 -> Vector Concatenate/27, Vector Concatenate/28
  Bit Slice17/1 -> Vector Concatenate/1, Vector Concatenate/2
  Bit Slice/1 -> Vector Concatenate/31, Vector Concatenate/32
  Bit Slice1/1 -> Vector Concatenate/29, Vector Concatenate/30
  Bit Slice7/1 -> Vector Concatenate/17, Vector Concatenate/18
  Vector Concatenate/1 -> Out1/1
  Bit Slice13/1 -> Vector Concatenate/9, Vector Concatenate/10
  Bit Slice9/1 -> Bit Slice/1, Bit Slice1/1, Bit Slice2/1, Bit Slice3/1, Bit Slice4/1, Bit Slice5/1, Bit Slice6/1, Bit Slice7/1
  Bit Slice11/1 -> Vector Concatenate/13, Vector Concatenate/14
  Bit Slice19/1 -> Bit Slice10/1, Bit Slice11/1, Bit Slice12/1, Bit Slice13/1, Bit Slice14/1, Bit Slice15/1, Bit Slice16/1, Bit Slice17/1
  u/1 -> Bit Slice9/1, Bit Slice19/1
  Bit Slice5/1 -> Vector Concatenate/21, Vector Concatenate/22
  Bit Slice6/1 -> Vector Concatenate/19, Vector Concatenate/20
  Bit Slice4/1 -> Vector Concatenate/23, Vector Concatenate/24
  Bit Slice10/1 -> Vector Concatenate/15, Vector Concatenate/16

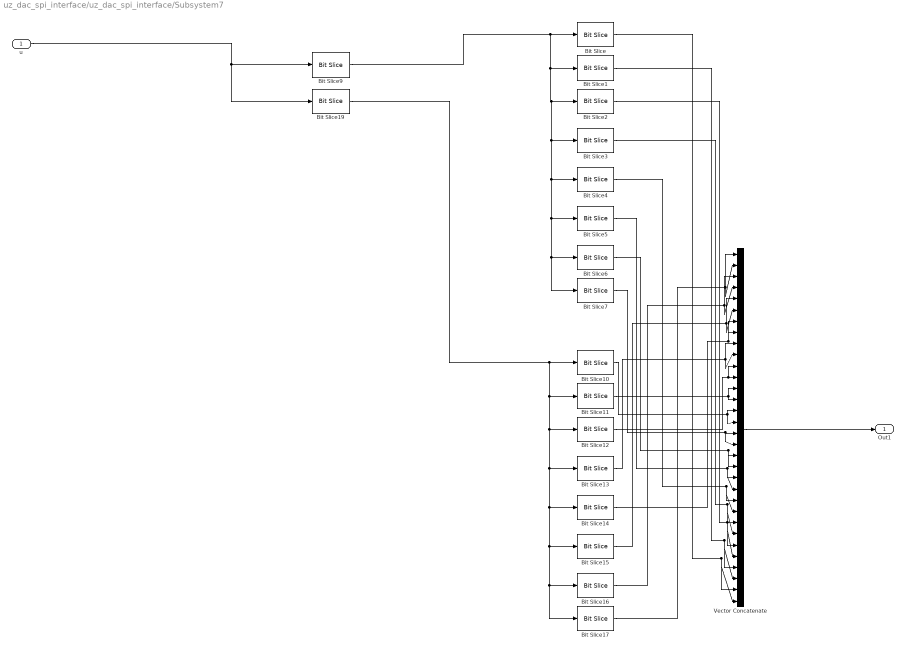
== system uz_dac_spi_interface/uz_dac_spi_interface/Subsystem7 ==
  u : Inport
  Bit Slice : hdlsllib/Logic and Bit Operations/Bit Slice  lidx=0  ridx=0
  Bit Slice1 : hdlsllib/Logic and Bit Operations/Bit Slice  lidx=1  ridx=1
  Bit Slice10 : hdlsllib/Logic and Bit Operations/Bit Slice  lidx=0  ridx=0
  Bit Slice11 : hdlsllib/Logic and Bit Operations/Bit Slice  lidx=1  ridx=1
  Bit Slice12 : hdlsllib/Logic and Bit Operations/Bit Slice  lidx=2  ridx=2
  Bit Slice13 : hdlsllib/Logic and Bit Operations/Bit Slice  lidx=3  ridx=3
  Bit Slice14 : hdlsllib/Logic and Bit Operations/Bit Slice  lidx=4  ridx=4
  Bit Slice15 : hdlsllib/Logic and Bit Operations/Bit Slice  lidx=5  ridx=5
  Bit Slice16 : hdlsllib/Logic and Bit Operations/Bit Slice  lidx=6  ridx=6
  Bit Slice17 : hdlsllib/Logic and Bit Operations/Bit Slice  lidx=7  ridx=7
  Bit Slice19 : hdlsllib/Logic and Bit Operations/Bit Slice  lidx=15  ridx=8
  Bit Slice2 : hdlsllib/Logic and Bit Operations/Bit Slice  lidx=2  ridx=2
  Bit Slice3 : hdlsllib/Logic and Bit Operations/Bit Slice  lidx=3  ridx=3
  Bit Slice4 : hdlsllib/Logic and Bit Operations/Bit Slice  lidx=4  ridx=4
  Bit Slice5 : hdlsllib/Logic and Bit Operations/Bit Slice  lidx=5  ridx=5
  Bit Slice6 : hdlsllib/Logic and Bit Operations/Bit Slice  lidx=6  ridx=6
  Bit Slice7 : hdlsllib/Logic and Bit Operations/Bit Slice  lidx=7  ridx=7
  Bit Slice9 : hdlsllib/Logic and Bit Operations/Bit Slice  lidx=7  ridx=0
  Vector Concatenate : Concatenate  NumInputs=32
  Out1 : Outport
  wires:
  Bit Slice15/1 -> Vector Concatenate/5, Vector Concatenate/6
  Bit Slice3/1 -> Vector Concatenate/25, Vector Concatenate/26
  Bit Slice14/1 -> Vector Concatenate/7, Vector Concatenate/8
  Bit Slice16/1 -> Vector Concatenate/3, Vector Concatenate/4
  Bit Slice12/1 -> Vector Concatenate/11, Vector Concatenate/12
  Bit Slice2/1 -> Vector Concatenate/27, Vector Concatenate/28
  Bit Slice17/1 -> Vector Concatenate/1, Vector Concatenate/2
  Bit Slice/1 -> Vector Concatenate/31, Vector Concatenate/32
  Bit Slice1/1 -> Vector Concatenate/29, Vector Concatenate/30
  Bit Slice7/1 -> Vector Concatenate/17, Vector Concatenate/18
  Vector Concatenate/1 -> Out1/1
  Bit Slice13/1 -> Vector Concatenate/9, Vector Concatenate/10
  Bit Slice9/1 -> Bit Slice/1, Bit Slice1/1, Bit Slice2/1, Bit Slice3/1, Bit Slice4/1, Bit Slice5/1, Bit Slice6/1, Bit Slice7/1
  Bit Slice11/1 -> Vector Concatenate/13, Vector Concatenate/14
  Bit Slice19/1 -> Bit Slice10/1, Bit Slice11/1, Bit Slice12/1, Bit Slice13/1, Bit Slice14/1, Bit Slice15/1, Bit Slice16/1, Bit Slice17/1
  u/1 -> Bit Slice9/1, Bit Slice19/1
  Bit Slice5/1 -> Vector Concatenate/21, Vector Concatenate/22
  Bit Slice6/1 -> Vector Concatenate/19, Vector Concatenate/20
  Bit Slice4/1 -> Vector Concatenate/23, Vector Concatenate/24
  Bit Slice10/1 -> Vector Concatenate/15, Vector Concatenate/16
